simulink model "untitled"  (R2016b)
settings: Solver=FixedStepAuto  StartTime=0.0  StopTime=20  FixedStep=0.0001  RelTol=1e-3
values from neighbouring files (symbols this model uses):
  K = Kf*R/Km+Ke    (= 4.8)    [momentFun.m]
undefined symbols (not defined in the file or in its folder): A, B, C
settings Model: Creator=texnoman  LastModifiedBy=root

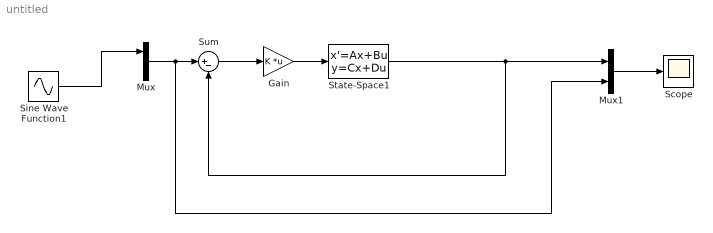
== system untitled ==
  Gain : Gain  Gain=K  Multiplication=Matrix(K*u)
  Mux : Mux  Inputs=3
  Mux1 : Mux  Inputs=2
  Scope : Scope
  Sine Wave Function1 : Sin  Amplitude=-5  Frequency=0.5  SampleTime=0
  State-Space1 : StateSpace  A=A  B=B  C=C  D=[0;0;0]  X0=[1;0;0]
  Sum : Sum  Inputs=|+-
  wires:
  Sum/1 -> Gain/1
  Mux/1 -> Mux1/2, Sum/1
  Mux1/1 -> Scope/1
  State-Space1/1 -> Sum/2, Mux1/1
  Sine Wave Function1/1 -> Mux/1
  Gain/1 -> State-Space1/1
